simulink model "Antriebsstrangmodell_V2"  (R2019a)
settings: Solver=FixedStepAuto  StartTime=0.0  StopTime=t_Simulation  FixedStep=dt  RelTol=1e-3
values from neighbouring files (symbols this model uses):
  cp_Luft = 1008.8    [Simulation_Antriebsstrangmodell_V2.m]
  eta_EMaschine_Break_M_EMaschine = flipud(KennfeldMaschine.M(:,1))'    [Simulation_Antriebsstrangmodell_V2.m]
  eta_EMaschine_Break_M_EMaschine_reku = -KennfeldMaschine.M(:,1)'    [Simulation_Antriebsstrangmodell_V2.m]
  eta_EMaschine_Break_n_EMaschine = KennfeldMaschine.n(end-1,:)    [Simulation_Antriebsstrangmodell_V2.m]
  eta_EMaschine_Break_n_EMaschine_reku = KennfeldMaschine.n(end-1,:)    [Simulation_Antriebsstrangmodell_V2.m]
  eta_EMaschine_Faktor_Volllast = 0.97    [Simulation_Antriebsstrangmodell_V2.m]
  eta_EMaschine_Table = flip(KennfeldMaschine.etages,1)    [Simulation_Antriebsstrangmodell_V2.m]
  eta_EMaschine_Table_reku = KennfeldMaschine.etages    [Simulation_Antriebsstrangmodell_V2.m]
  h_WC_pumpoff = Nu_WC*lam_WC/dh_WC    [Simulation_Antriebsstrangmodell_V2.m]
  h_WC_pumpon = Nu_WC*lam_WC/dh_WC    [Simulation_Antriebsstrangmodell_V2.m]
  lam_Luft = 0.028592    [Simulation_Antriebsstrangmodell_V2.m]
  M_EMaschine_max = zeros(2,numel(eta_EMaschine_Break_n_EMaschine))    [Simulation_Antriebsstrangmodell_V2.m]
  nue_Luft = 19.230034390524e-6    (= 1.92300343905e-05)    [Simulation_Antriebsstrangmodell_V2.m]
  pump_start_limit = 273.15 + 33    (= 306.15)    [Simulation_Antriebsstrangmodell_V2.m]
  rho_Luft = 1.0468    [Simulation_Antriebsstrangmodell_V2.m]
  share_EMaschine_Ummagnet_reku_Table = ser.gen.share_Ummagnetisierungsverluste    [Simulation_Antriebsstrangmodell_V2.m]
  share_EMaschine_Ummagnet_Table = ser.mot.share_Ummagnetisierungsverluste    [Simulation_Antriebsstrangmodell_V2.m]
  share_EMaschine_Wicklung_reku_Table = ser.gen.share_Wicklungsverluste    [Simulation_Antriebsstrangmodell_V2.m]
  share_EMaschine_Wicklung_Table = ser.mot.share_Wicklungsverluste    [Simulation_Antriebsstrangmodell_V2.m]
  share_EMaschine_WirkMech_reku_Table = ser.gen.share_WirkmechVerluste    [Simulation_Antriebsstrangmodell_V2.m]
  share_EMaschine_WirkMech_Table = ser.mot.share_WirkmechVerluste    [Simulation_Antriebsstrangmodell_V2.m]
  share_EMaschine_WirkZus_reku_Table = ser.gen.share_WirkZusVerl    [Simulation_Antriebsstrangmodell_V2.m]
  share_EMaschine_WirkZus_Table = ser.mot.share_WirkZusVerl    [Simulation_Antriebsstrangmodell_V2.m]
  t_Simulation = 60*60    (= 3600)    [Simulation_Antriebsstrangmodell_V2.m]
  T_Start_Coolant = 273.15 + 25    (= 298.15)    [Simulation_Antriebsstrangmodell_V2.m]
  T_Start_EMaschine = 273.15 + 25    (= 298.15)    [Simulation_Antriebsstrangmodell_V2.m]
  Verlustleistung_Fit = 4    [Simulation_Antriebsstrangmodell_V2.m]
undefined symbols (not defined in the file or in its folder): Anteil_Stator, D_2a, delta, m_ER, m_RSL, m_RTO, m_RYO, m_SSL, m_STO, m_SYO, m_WH, v_EC_corr, v_ER_corr, v_WH_corr
libraries: fl_lib x72, nesl_utility x26, SimscapeCustomBlocks_lib x8, simulink x3
(part 2 of 2)

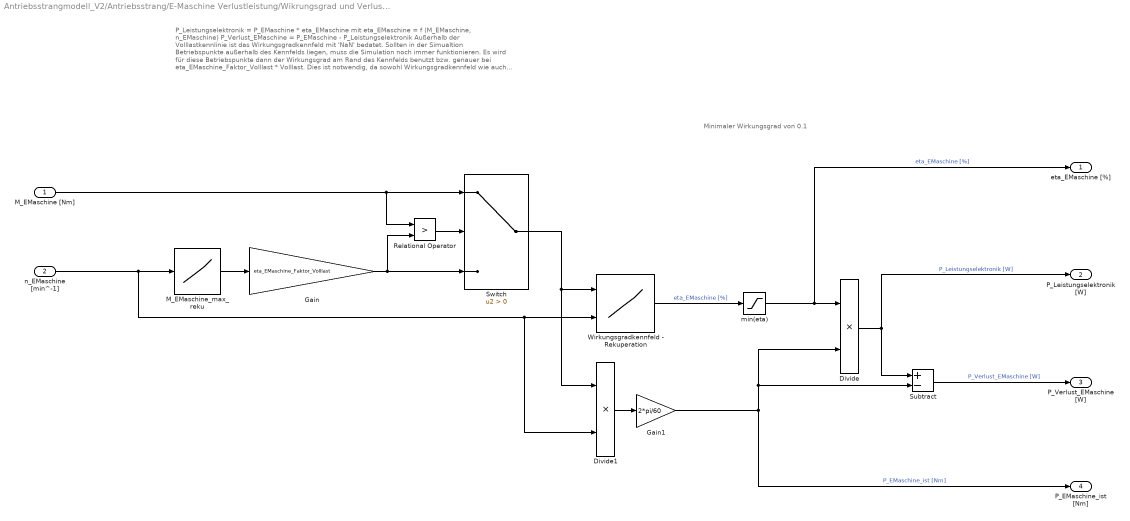
== system Antriebsstrangmodell_V2/Antriebsstrang/E-Maschine Verlustleistung/Wikrungsgrad und Verlustleistung - Rekuperation ==
  note: Minimaler Wirkungsgrad von 0.1
  note: P_Leistungselektronik = P_EMaschine * eta_EMaschine
      |
      | mit eta_EMaschine = f (M_EMaschine, n_EMaschine)
      |
      | P_Verlust_EMaschine = P_EMaschine - P_Leistungselektronik
      |
      | Außerhalb der Volllastkennlinie ist das Wirkungsgradkennfeld mit 'NaN' bedatet. Sollten in der Simualtion Betriebspunkte außerhalb des Kennfelds liegen, muss die Simulation noch immer funktionieren. Es wird für diese Betriebspunkte dann der Wirkungsgrad am Rand des Kennfelds benutzt bzw. genauer bei eta_EMaschine_Faktor_Volllast * Volllast. Dies ist notwendig, da sowohl Wirkungsgradkennfeld wie auch Lookup Table nicht stetig sind und somit zwischen Stützstellen interpolieren müssen. Dies kann dazu führen, dass ein Wert, der auf der Volllastlinie sitzt, in 'NaN' im Wirkungsgradkennfeld resultiert. Um dies zu vermeiden, wird mit eta_EMaschine_Faktor_Volllast * Volllast gerechnet, wenn Betriebspunkte außerhalb des Kennfelds liegen, um 'NaN' Wirkungsgrade zu vermeiden. eta_EMaschine_Faktor_Volllast ist stark abh. von der Güte (Abstand der Stützstellen) des Wirkungsgradkennfeldes.
  M_EMaschine [Nm] : Inport
  n_EMaschine [min^-1] : Inport  Port=2
  Divide : Product  Inputs=**
  Divide1 : Product  Inputs=**
  Gain : Gain  Gain=eta_EMaschine_Faktor_Volllast
  Gain1 : Gain  Gain=2*pi/60
  M_EMaschine_max_reku : Lookup_n-D  NumberOfTableDimensions=1  BreakpointsForDimension1=[-15,1700,2050,3400,4050,6100]  BeginIndexSearchUsingPreviousIndexResult=on  Table=[0.44,-52,-51,-37.5,-33,-27.25]  ExtrapMethod=Clip  UseLastTableValue=on  InternalRulePriority=Speed  RndMeth=Simplest  InputSameDT=on
  Relational Operator : RelationalOperator  Operator=>  OutDataTypeStr=boolean  RndMeth=Simplest
  Subtract : Sum  Inputs=+-
  Switch : Switch  Criteria=u2 > Threshold
  Wirkungsgradkennfeld - Rekuperation : Lookup_n-D  BreakpointsForDimension1=eta_EMaschine_Break_M_EMaschine_reku  BreakpointsForDimension2=eta_EMaschine_Break_n_EMaschine_reku  BeginIndexSearchUsingPreviousIndexResult=on  Table=eta_EMaschine_Table_reku  ExtrapMethod=Clip  UseLastTableValue=on  InternalRulePriority=Speed  RndMeth=Simplest  InputSameDT=on
  min(eta) : Saturate  UpperLimit=inf  LowerLimit=0.1
  eta_EMaschine [%] : Outport
  P_Leistungselektronik [W] : Outport  Port=2
  P_Verlust_EMaschine [W] : Outport  Port=3
  P_EMaschine_ist [Nm] : Outport  Port=4
  wires:
  Relational Operator/1 -> Switch/2
  Switch/1 -> Divide1/1, Wirkungsgradkennfeld - Rekuperation/1
  Subtract/1 -> P_Verlust_EMaschine [W]/1  "P_Verlust_EMaschine [W]"
  n_EMaschine [min^-1]/1 -> Divide1/2, Wirkungsgradkennfeld - Rekuperation/2, M_EMaschine_max_reku/1
  Wirkungsgradkennfeld - Rekuperation/1 -> min(eta)/1  "eta_EMaschine [%]"
  Gain/1 -> Relational Operator/2, Switch/3
  min(eta)/1 -> eta_EMaschine [%]/1, Divide/1  "eta_EMaschine [%]"
  M_EMaschine_max_reku/1 -> Gain/1
  M_EMaschine [Nm]/1 -> Switch/1, Relational Operator/1
  Divide/1 -> P_Leistungselektronik [W]/1, Subtract/1  "P_Leistungselektronik [W]"
  Divide1/1 -> Gain1/1
  Gain1/1 -> P_EMaschine_ist [Nm]/1, Subtract/2, Divide/2  "P_EMaschine_ist [Nm]"

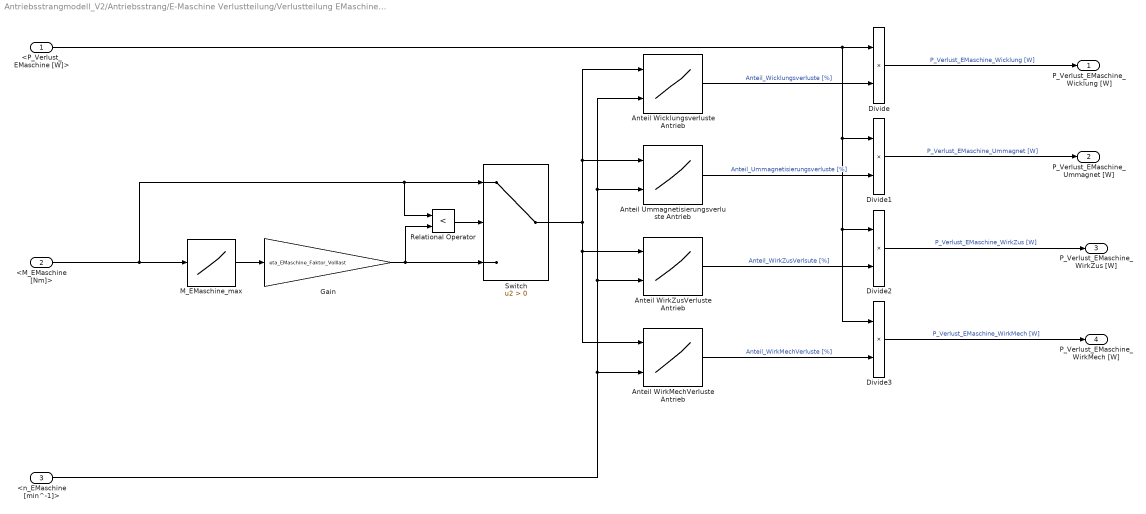
== system Antriebsstrangmodell_V2/Antriebsstrang/E-Maschine Verlustteilung/Verlustteilung EMaschine - Antrieb ==
  <P_Verlust_EMaschine [W]> : Inport
  <M_EMaschine [Nm]> : Inport  Port=2
  <n_EMaschine [min^-1]> : Inport  Port=3
  Anteil Ummagnetisierungsverluste Antrieb : Lookup_n-D  BreakpointsForDimension1=eta_EMaschine_Break_M_EMaschine  BreakpointsForDimension2=eta_EMaschine_Break_n_EMaschine  BeginIndexSearchUsingPreviousIndexResult=on  Table=share_EMaschine_Ummagnet_Table  ExtrapMethod=Clip  UseLastTableValue=on  InternalRulePriority=Speed  RndMeth=Simplest  InputSameDT=on
  Anteil Wicklungsverluste Antrieb : Lookup_n-D  BreakpointsForDimension1=eta_EMaschine_Break_M_EMaschine  BreakpointsForDimension2=eta_EMaschine_Break_n_EMaschine  BeginIndexSearchUsingPreviousIndexResult=on  Table=share_EMaschine_Wicklung_Table  ExtrapMethod=Clip  UseLastTableValue=on  InternalRulePriority=Speed  RndMeth=Simplest  InputSameDT=on
  Anteil WirkMechVerluste Antrieb : Lookup_n-D  BreakpointsForDimension1=eta_EMaschine_Break_M_EMaschine  BreakpointsForDimension2=eta_EMaschine_Break_n_EMaschine  BeginIndexSearchUsingPreviousIndexResult=on  Table=share_EMaschine_WirkMech_Table  ExtrapMethod=Clip  UseLastTableValue=on  InternalRulePriority=Speed  RndMeth=Simplest  InputSameDT=on
  Anteil WirkZusVerluste Antrieb : Lookup_n-D  BreakpointsForDimension1=eta_EMaschine_Break_M_EMaschine  BreakpointsForDimension2=eta_EMaschine_Break_n_EMaschine  BeginIndexSearchUsingPreviousIndexResult=on  Table=share_EMaschine_WirkZus_Table  ExtrapMethod=Clip  UseLastTableValue=on  InternalRulePriority=Speed  RndMeth=Simplest  InputSameDT=on
  Divide{,1..3} (4 alike) : Product  Inputs=**
  Gain : Gain  Gain=eta_EMaschine_Faktor_Volllast
  M_EMaschine_max : Lookup_n-D  NumberOfTableDimensions=1  BreakpointsForDimension1=M_EMaschine_max(1,:)  BeginIndexSearchUsingPreviousIndexResult=on  Table=M_EMaschine_max(2,:)  ExtrapMethod=Clip  UseLastTableValue=on  InternalRulePriority=Speed  RndMeth=Simplest  InputSameDT=on
  Relational Operator : RelationalOperator  Operator=<  OutDataTypeStr=boolean  RndMeth=Simplest
  Switch : Switch  Criteria=u2 > Threshold
  P_Verlust_EMaschine_Wicklung [W] : Outport
  P_Verlust_EMaschine_Ummagnet [W] : Outport  Port=2
  P_Verlust_EMaschine_WirkZus [W] : Outport  Port=3
  P_Verlust_EMaschine_WirkMech [W] : Outport  Port=4
  wires:
  Anteil Wicklungsverluste Antrieb/1 -> Divide/2  "Anteil_Wicklungsverluste [%]"
  M_EMaschine_max/1 -> Gain/1
  <n_EMaschine [min^-1]>/1 -> Anteil Wicklungsverluste Antrieb/2, Anteil Ummagnetisierungsverluste Antrieb/2, Anteil WirkZusVerluste Antrieb/2, Anteil WirkMechVerluste Antrieb/2
  <P_Verlust_EMaschine [W]>/1 -> Divide3/1, Divide2/1, Divide1/1, Divide/1
  Gain/1 -> Relational Operator/2, Switch/3
  Anteil WirkMechVerluste Antrieb/1 -> Divide3/2  "Anteil_WirkMechVerluste [%]"
  Switch/1 -> Anteil WirkMechVerluste Antrieb/1, Anteil WirkZusVerluste Antrieb/1, Anteil Wicklungsverluste Antrieb/1, Anteil Ummagnetisierungsverluste Antrieb/1
  Relational Operator/1 -> Switch/2
  Divide/1 -> P_Verlust_EMaschine_Wicklung [W]/1  "P_Verlust_EMaschine_Wicklung [W]"
  Anteil Ummagnetisierungsverluste Antrieb/1 -> Divide1/2  "Anteil_Ummagnetisierungsverluste [%]"
  Anteil WirkZusVerluste Antrieb/1 -> Divide2/2  "Anteil_WirkZusVerlsute [%]"
  Divide3/1 -> P_Verlust_EMaschine_WirkMech [W]/1  "P_Verlust_EMaschine_WirkMech [W]"
  Divide1/1 -> P_Verlust_EMaschine_Ummagnet [W]/1  "P_Verlust_EMaschine_Ummagnet [W]"
  Divide2/1 -> P_Verlust_EMaschine_WirkZus [W]/1  "P_Verlust_EMaschine_WirkZus [W]"
  <M_EMaschine [Nm]>/1 -> Relational Operator/1, Switch/1, M_EMaschine_max/1

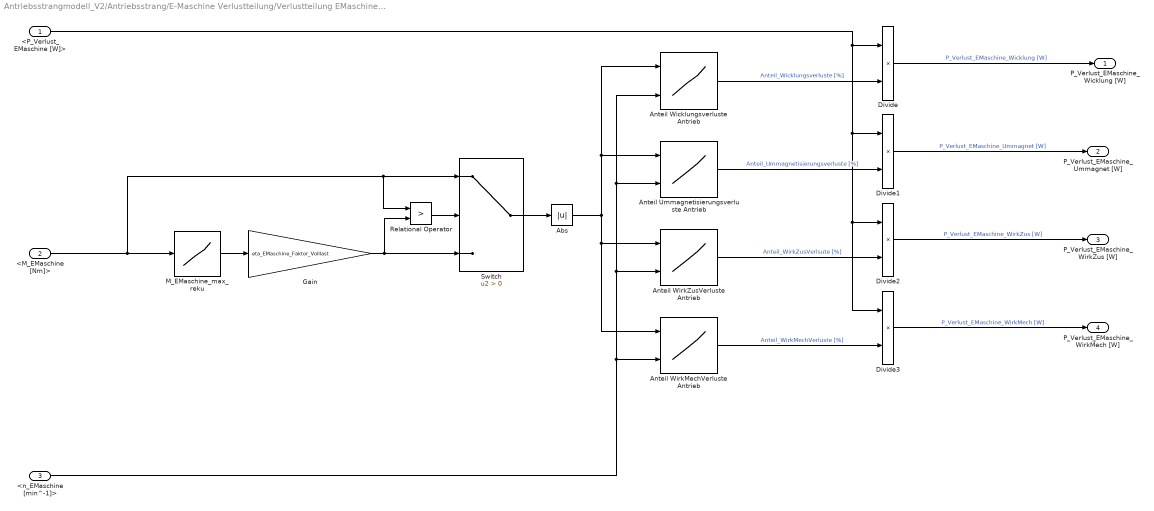
== system Antriebsstrangmodell_V2/Antriebsstrang/E-Maschine Verlustteilung/Verlustteilung EMaschine - Rekuperation ==
  <P_Verlust_EMaschine [W]> : Inport
  <M_EMaschine [Nm]> : Inport  Port=2
  <n_EMaschine [min^-1]> : Inport  Port=3
  Abs : Abs
  Anteil Ummagnetisierungsverluste Antrieb : Lookup_n-D  BreakpointsForDimension1=eta_EMaschine_Break_M_EMaschine  BreakpointsForDimension2=eta_EMaschine_Break_n_EMaschine  BeginIndexSearchUsingPreviousIndexResult=on  Table=share_EMaschine_Ummagnet_reku_Table  ExtrapMethod=Clip  UseLastTableValue=on  InternalRulePriority=Speed  RndMeth=Simplest  InputSameDT=on
  Anteil Wicklungsverluste Antrieb : Lookup_n-D  BreakpointsForDimension1=eta_EMaschine_Break_M_EMaschine  BreakpointsForDimension2=eta_EMaschine_Break_n_EMaschine  BeginIndexSearchUsingPreviousIndexResult=on  Table=share_EMaschine_Wicklung_reku_Table  ExtrapMethod=Clip  UseLastTableValue=on  InternalRulePriority=Speed  RndMeth=Simplest  InputSameDT=on
  Anteil WirkMechVerluste Antrieb : Lookup_n-D  BreakpointsForDimension1=eta_EMaschine_Break_M_EMaschine  BreakpointsForDimension2=eta_EMaschine_Break_n_EMaschine  BeginIndexSearchUsingPreviousIndexResult=on  Table=share_EMaschine_WirkMech_reku_Table  ExtrapMethod=Clip  UseLastTableValue=on  InternalRulePriority=Speed  RndMeth=Simplest  InputSameDT=on
  Anteil WirkZusVerluste Antrieb : Lookup_n-D  BreakpointsForDimension1=eta_EMaschine_Break_M_EMaschine  BreakpointsForDimension2=eta_EMaschine_Break_n_EMaschine  BeginIndexSearchUsingPreviousIndexResult=on  Table=share_EMaschine_WirkZus_reku_Table  ExtrapMethod=Clip  UseLastTableValue=on  InternalRulePriority=Speed  RndMeth=Simplest  InputSameDT=on
  Divide{,1..3} (4 alike) : Product  Inputs=**
  Gain : Gain  Gain=eta_EMaschine_Faktor_Volllast
  M_EMaschine_max_reku : Lookup_n-D  NumberOfTableDimensions=1  BreakpointsForDimension1=[-15,1700,2050,3400,4050,6100]  BeginIndexSearchUsingPreviousIndexResult=on  Table=[0.44,-52,-51,-37.5,-33,-27.25]  ExtrapMethod=Clip  UseLastTableValue=on  InternalRulePriority=Speed  RndMeth=Simplest  InputSameDT=on
  Relational Operator : RelationalOperator  Operator=>  OutDataTypeStr=boolean  RndMeth=Simplest
  Switch : Switch  Criteria=u2 > Threshold
  P_Verlust_EMaschine_Wicklung [W] : Outport
  P_Verlust_EMaschine_Ummagnet [W] : Outport  Port=2
  P_Verlust_EMaschine_WirkZus [W] : Outport  Port=3
  P_Verlust_EMaschine_WirkMech [W] : Outport  Port=4
  wires:
  Anteil Wicklungsverluste Antrieb/1 -> Divide/2  "Anteil_Wicklungsverluste [%]"
  M_EMaschine_max_reku/1 -> Gain/1
  <n_EMaschine [min^-1]>/1 -> Anteil Wicklungsverluste Antrieb/2, Anteil Ummagnetisierungsverluste Antrieb/2, Anteil WirkZusVerluste Antrieb/2, Anteil WirkMechVerluste Antrieb/2
  <P_Verlust_EMaschine [W]>/1 -> Divide3/1, Divide2/1, Divide1/1, Divide/1
  Gain/1 -> Relational Operator/2, Switch/3
  Anteil WirkMechVerluste Antrieb/1 -> Divide3/2  "Anteil_WirkMechVerluste [%]"
  Switch/1 -> Abs/1
  Relational Operator/1 -> Switch/2
  Divide/1 -> P_Verlust_EMaschine_Wicklung [W]/1  "P_Verlust_EMaschine_Wicklung [W]"
  Anteil Ummagnetisierungsverluste Antrieb/1 -> Divide1/2  "Anteil_Ummagnetisierungsverluste [%]"
  Anteil WirkZusVerluste Antrieb/1 -> Divide2/2  "Anteil_WirkZusVerlsute [%]"
  Divide3/1 -> P_Verlust_EMaschine_WirkMech [W]/1  "P_Verlust_EMaschine_WirkMech [W]"
  Divide1/1 -> P_Verlust_EMaschine_Ummagnet [W]/1  "P_Verlust_EMaschine_Ummagnet [W]"
  Divide2/1 -> P_Verlust_EMaschine_WirkZus [W]/1  "P_Verlust_EMaschine_WirkZus [W]"
  <M_EMaschine [Nm]>/1 -> M_EMaschine_max_reku/1, Relational Operator/1, Switch/1
  Abs/1 -> Anteil WirkMechVerluste Antrieb/1, Anteil WirkZusVerluste Antrieb/1, Anteil Wicklungsverluste Antrieb/1, Anteil Ummagnetisierungsverluste Antrieb/1

== system Antriebsstrangmodell_V2/Antriebsstrang/E-Maschine Thermik/Thermisches Netzwerk/Subsystem ==

== system Antriebsstrangmodell_V2/Antriebsstrang/E-Maschine Thermik/Thermisches Netzwerk/Subsystem1 ==

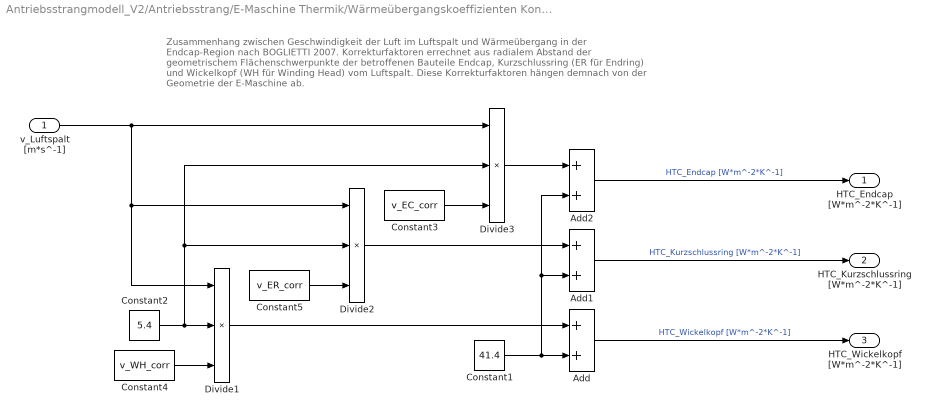
== system Antriebsstrangmodell_V2/Antriebsstrang/E-Maschine Thermik/Wärmeübergangskoeffizienten Konvektion Luftspalt und Endcap-Luft/Endcap-Luft-Konvektion ==
  note: Zusammenhang zwischen Geschwindigkeit der Luft im Luftspalt und Wärmeübergang in der Endcap-Region nach BOGLIETTI 2007.
      | Korrekturfaktoren errechnet aus radialem Abstand der geometrischem Flächenschwerpunkte der betroffenen Bauteile Endcap,
      | Kurzschlussring (ER für Endring) und Wickelkopf (WH für Winding Head) vom Luftspalt.
      | Diese Korrekturfaktoren hängen demnach von der Geometrie der E-Maschine ab.
  v_Luftspalt [m*s^-1] : Inport
  Add : Sum
  Add1 : Sum
  Add2 : Sum
  Constant1 : Constant  Value=41.4
  Constant2 : Constant  Value=5.4
  Constant3 : Constant  Value=v_EC_corr
  Constant4 : Constant  Value=v_WH_corr
  Constant5 : Constant  Value=v_ER_corr
  Divide1 : Product  Inputs=***
  Divide2 : Product  Inputs=***
  Divide3 : Product  Inputs=***
  HTC_Endcap [W*m^-2*K^-1] : Outport
  HTC_Kurzschlussring [W*m^-2*K^-1] : Outport  Port=2
  HTC_Wickelkopf [W*m^-2*K^-1] : Outport  Port=3
  wires:
  Add/1 -> HTC_Wickelkopf [W*m^-2*K^-1]/1  "HTC_Wickelkopf [W*m^-2*K^-1]"
  Constant3/1 -> Divide3/3
  Divide3/1 -> Add2/1
  v_Luftspalt [m*s^-1]/1 -> Divide1/1, Divide2/1, Divide3/1
  Constant2/1 -> Divide1/2, Divide3/2, Divide2/2
  Constant1/1 -> Add/2, Add1/2, Add2/2
  Constant4/1 -> Divide1/3
  Constant5/1 -> Divide2/3
  Divide2/1 -> Add1/1
  Divide1/1 -> Add/1
  Add1/1 -> HTC_Kurzschlussring [W*m^-2*K^-1]/1  "HTC_Kurzschlussring [W*m^-2*K^-1]"
  Add2/1 -> HTC_Endcap [W*m^-2*K^-1]/1  "HTC_Endcap [W*m^-2*K^-1]"

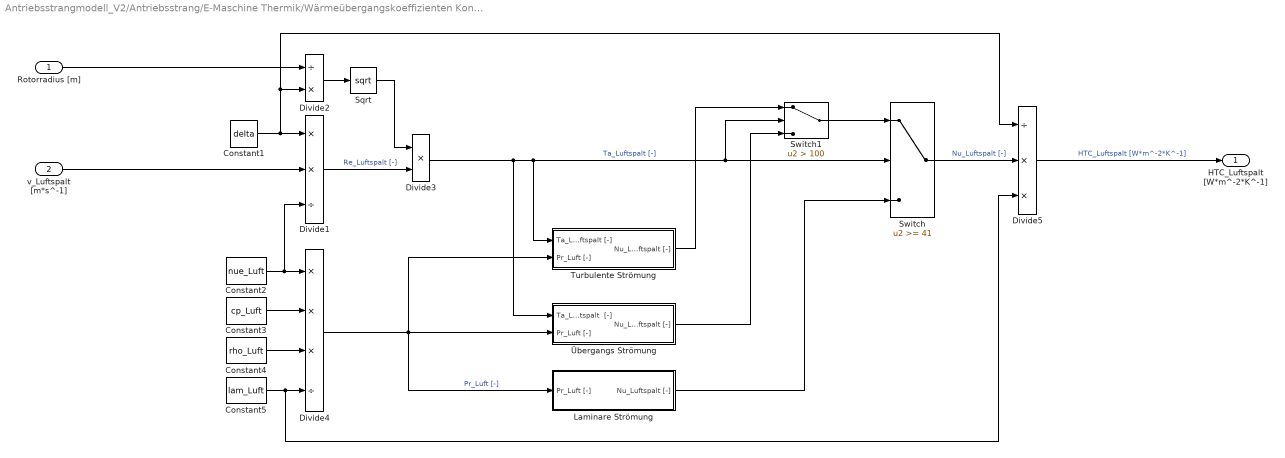
== system Antriebsstrangmodell_V2/Antriebsstrang/E-Maschine Thermik/Wärmeübergangskoeffizienten Konvektion Luftspalt und Endcap-Luft/Luftspalt-Konvektion ==
  Rotorradius [m] : Inport
  v_Luftspalt [m*s^-1] : Inport  Port=2
  Constant1 : Constant  Value=delta
  Constant2 : Constant  Value=nue_Luft
  Constant3 : Constant  Value=cp_Luft
  Constant4 : Constant  Value=rho_Luft
  Constant5 : Constant  Value=lam_Luft
  Divide1 : Product  Inputs=**/
  Divide2 : Product  Inputs=/*
  Divide3 : Product  Inputs=**
  Divide4 : Product  Inputs=***/
  Divide5 : Product  Inputs=/**
  Laminare Strömung : Subsystem
  Sqrt : Sqrt  SaturateOnIntegerOverflow=on
  Switch : Switch  Threshold=41
  Switch1 : Switch  Criteria=u2 > Threshold  Threshold=100
  Turbulente Strömung : Subsystem
  Übergangs Strömung : Subsystem
  HTC_Luftspalt [W*m^-2*K^-1] : Outport
  wires:
  Divide3/1 -> Switch1/2, Switch/2, Turbulente Strömung/1(Ta_Luftspalt [-]), Übergangs Strömung/1(Ta_Luftspalt  [-])  "Ta_Luftspalt [-]"
  Constant4/1 -> Divide4/3
  Divide4/1 -> Übergangs Strömung/2(Pr_Luft [-]), Laminare Strömung/1(Pr_Luft [-]), Turbulente Strömung/2(Pr_Luft [-])  "Pr_Luft [-]"
  Rotorradius [m]/1 -> Divide2/1
  Constant2/1 -> Divide1/3, Divide4/1
  Laminare Strömung/1(Nu_Luftspalt [-]) -> Switch/3
  Turbulente Strömung/1(Nu_Luftspalt [-]) -> Switch1/1
  Constant1/1 -> Divide5/1, Divide2/2, Divide1/1
  Übergangs Strömung/1(Nu_Luftspalt [-]) -> Switch1/3
  Constant5/1 -> Divide5/3, Divide4/4
  Divide1/1 -> Divide3/2  "Re_Luftspalt [-]"
  Switch1/1 -> Switch/1
  Switch/1 -> Divide5/2  "Nu_Luftspalt [-]"
  Sqrt/1 -> Divide3/1
  v_Luftspalt [m*s^-1]/1 -> Divide1/2
  Divide5/1 -> HTC_Luftspalt [W*m^-2*K^-1]/1  "HTC_Luftspalt [W*m^-2*K^-1]"
  Constant3/1 -> Divide4/2
  Divide2/1 -> Sqrt/1

== system Antriebsstrangmodell_V2/Antriebsstrang/E-Maschine Thermik/Wärmeübergangskoeffizienten Konvektion Luftspalt und Endcap-Luft/Luftspalt-Konvektion/Laminare Strömung ==
  Pr_Luft [-] : Inport
  Constant6 : Constant  Value=41
  Constant7 : Constant  Value=0.63
  Constant8 : Constant  Value=0.202
  Constant9 : Constant  Value=0.27
  Divide5 : Product  Inputs=***
  Math Function : Math  Operator=pow  SaturateOnIntegerOverflow=on
  Math Function1 : Math  Operator=pow  SaturateOnIntegerOverflow=on
  Nu_Luftspalt [-] : Outport
  wires:
  Constant6/1 -> Math Function/1
  Constant7/1 -> Math Function/2
  Math Function/1 -> Divide5/2
  Math Function1/1 -> Divide5/3
  Constant9/1 -> Math Function1/2
  Pr_Luft [-]/1 -> Math Function1/1
  Constant8/1 -> Divide5/1
  Divide5/1 -> Nu_Luftspalt [-]/1  "Nu_Luftspalt [-]"

== system Antriebsstrangmodell_V2/Antriebsstrang/E-Maschine Thermik/Wärmeübergangskoeffizienten Konvektion Luftspalt und Endcap-Luft/Luftspalt-Konvektion/Turbulente Strömung ==
  Ta_Luftspalt [-] : Inport
  Pr_Luft [-] : Inport  Port=2
  Constant7 : Constant  Value=0.5
  Constant8 : Constant  Value=0.386
  Constant9 : Constant  Value=0.27
  Divide5 : Product  Inputs=***
  Math Function : Math  Operator=pow  SaturateOnIntegerOverflow=on
  Math Function1 : Math  Operator=pow  SaturateOnIntegerOverflow=on
  Nu_Luftspalt [-] : Outport
  wires:
  Ta_Luftspalt [-]/1 -> Math Function/1
  Constant7/1 -> Math Function/2
  Math Function/1 -> Divide5/2
  Math Function1/1 -> Divide5/3
  Constant9/1 -> Math Function1/2
  Pr_Luft [-]/1 -> Math Function1/1
  Constant8/1 -> Divide5/1
  Divide5/1 -> Nu_Luftspalt [-]/1  "Nu_Luftspalt [-]"

== system Antriebsstrangmodell_V2/Antriebsstrang/E-Maschine Thermik/Wärmeübergangskoeffizienten Konvektion Luftspalt und Endcap-Luft/Luftspalt-Konvektion/Übergangs Strömung ==
  Ta_Luftspalt  [-] : Inport
  Pr_Luft [-] : Inport  Port=2
  Constant7 : Constant  Value=0.63
  Constant8 : Constant  Value=0.202
  Constant9 : Constant  Value=0.27
  Divide5 : Product  Inputs=***
  Math Function : Math  Operator=pow  SaturateOnIntegerOverflow=on
  Math Function1 : Math  Operator=pow  SaturateOnIntegerOverflow=on
  Nu_Luftspalt [-] : Outport
  wires:
  Ta_Luftspalt  [-]/1 -> Math Function/1
  Constant7/1 -> Math Function/2
  Math Function/1 -> Divide5/2
  Math Function1/1 -> Divide5/3
  Constant9/1 -> Math Function1/2
  Pr_Luft [-]/1 -> Math Function1/1
  Constant8/1 -> Divide5/1
  Divide5/1 -> Nu_Luftspalt [-]/1  "Nu_Luftspalt [-]"
